simulink model "model_linear_observador"  (R2022a)
settings: Solver=VariableStepAuto  StartTime=0  StopTime=100  RelTol=1e-3
values from neighbouring files (symbols this model uses):
  A = [ 0 1 0  0 ... (first row only)    [ball_and_beam_pfc.m]
  amplitude_entrada = 0.05    [ball_and_beam_pfc.m]
  B = [0 ... (first row only)    [ball_and_beam_pfc.m]
  bool_degrau = 1    [ball_and_beam_pfc.m]
  C = [0 0 1 0]    [ball_and_beam_pfc.m]
  k_seguimento = K_nulo(1:4)    [ball_and_beam_pfc.m]
  ki_seguimento = K_nulo(5)    [ball_and_beam_pfc.m]
  L = 0.425    [ball_and_beam_pfc.m]    (also in nonlinear_ball_and_beam.m)
  L_observer = inv(T)*Lchp    [ball_and_beam_pfc.m]
libraries: vrlib x3
settings Model: Creator=Notebook_Artur  LastModifiedBy=Notebook_Artur

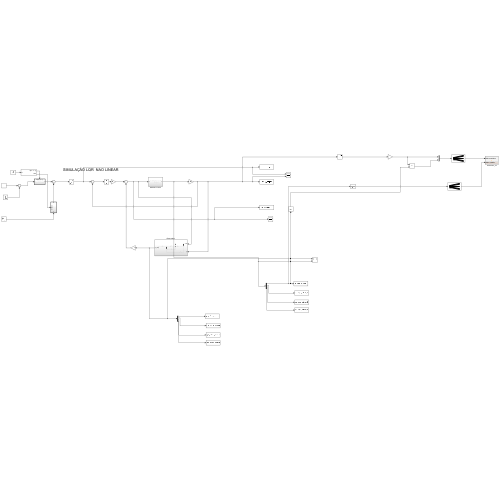
[thumbnail: Simulink's stored preview of the top-level diagram]
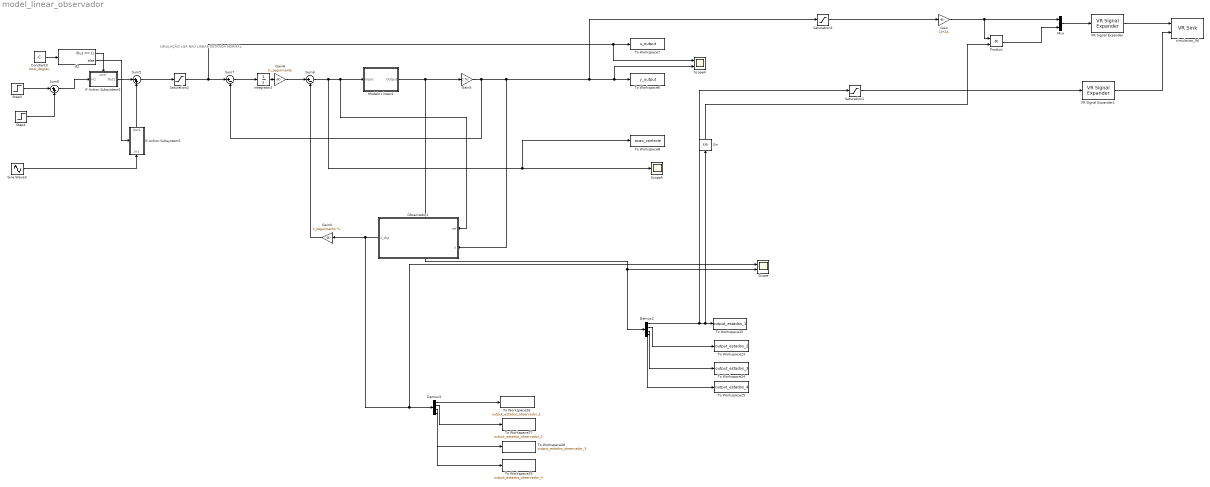
== system model_linear_observador ==
  note: SIMULAÇÃO LQR NAO LINEAR ENTRADA NORMAL
  Constant3 : Constant  Value=bool_degrau
  Demux2 : Demux
  Demux3 : Demux
  Gain : Gain  Gain=13*2/L
  Gain4 : Gain  Gain=k_seguimento  Multiplication=Matrix(K*u)
  Gain5 : Gain  Gain=C  Multiplication=Matrix(K*u)
  Gain6 : Gain  Gain=ki_seguimento
  If Action Subsystem5 : Subsystem  TreatAsAtomicUnit=on
  If Action Subsystem6 : Subsystem  TreatAsAtomicUnit=on
  If2 : If  IfExpression=u1 == 1
  Integrator2 : Integrator
  Modelo Linear2 : Subsystem
  Mux : Mux  Inputs=2
  Observador1 : Subsystem
  Product : Product
  Saturation1 : Saturate  UpperLimit=0.8  LowerLimit=-0.8
  Saturation2 : Saturate  UpperLimit=L/2  LowerLimit=-L/2
  Saturation3 : Saturate  UpperLimit=L/2  LowerLimit=0
  Scope : Scope  NumInputPorts=2
  Scope4 : Scope  NumInputPorts=2
  Scope5 : Scope
  Sin : Trigonometry
  Sine Wave3 : Sin  Amplitude=amplitude_entrada  Frequency=0.1  SampleTime=0
  Step3 : Step  After=amplitude_entrada  SampleTime=0
  Step4 : Step  Time=100  After=-2*amplitude_entrada  SampleTime=0
  Sum5 : Sum  Inputs=|++
  Sum6 : Sum  Inputs=|+-
  Sum7 : Sum  Inputs=|+-
  Sum8 : Sum  Inputs=|++
  To Workspace15 : ToWorkspace  VariableName=output_estados_1  SaveFormat=Timeseries  SampleTime=-1
  To Workspace23 : ToWorkspace  VariableName=output_estados_2  SaveFormat=Timeseries  SampleTime=-1
  To Workspace24 : ToWorkspace  VariableName=output_estados_3  SaveFormat=Timeseries  SampleTime=-1
  To Workspace25 : ToWorkspace  VariableName=output_estados_4  SaveFormat=Timeseries  SampleTime=-1
  To Workspace26 : ToWorkspace  VariableName=output_estados_observador_1  SaveFormat=Timeseries  SampleTime=-1
  To Workspace27 : ToWorkspace  VariableName=output_estados_observador_2  SaveFormat=Timeseries  SampleTime=-1
  To Workspace28 : ToWorkspace  VariableName=output_estados_observador_3  SaveFormat=Timeseries  SampleTime=-1
  To Workspace29 : ToWorkspace  VariableName=output_estados_observador_4  SaveFormat=Timeseries  SampleTime=-1
  To Workspace6 : ToWorkspace  VariableName=y_output  SaveFormat=Timeseries  SampleTime=-1
  To Workspace7 : ToWorkspace  VariableName=u_output  SaveFormat=Timeseries  SampleTime=-1
  To Workspace8 : ToWorkspace  VariableName=acao_controle  SaveFormat=Timeseries  SampleTime=-1
  VR Signal Expander : vrlib/VR Signal Expander  outwidth=3  outidx=[1 3]
  VR Signal Expander1 : vrlib/VR Signal Expander  outwidth=4  outidx=[4]
  simulacao_3d : vrlib/VR Sink  InstantiateOnLoad=on  SampleTime=0.1  ViewEnable=on  RemoteChange=off  RemoteView=off  FieldsWritten=Ball.translation.3.1.1.double#beam.rotation.4.1.1.double  WorldFileName=3d_ball_and_beam4.x3d  AutoView=on  VideoDimensions=[]  AllowVariableSize=off
  wires:
  If Action Subsystem6/1(Out1) -> Sum5/1
  Demux2/2 -> To Workspace23/1
  Demux3/2 -> To Workspace27/1
  Integrator2/1 -> Gain6/1
  If2/2 -> If Action Subsystem5/Action
  Demux2/3 -> To Workspace24/1
  Demux3/4 -> To Workspace29/1
  Demux3/3 -> To Workspace28/1
  If2/1 -> If Action Subsystem6/Action
  Modelo Linear2/1(Output) -> Gain5/1, Demux2/1, Scope/2
  Gain6/1 -> Sum6/1
  If Action Subsystem5/1(Out1) -> Sum5/2
  Demux2/4 -> To Workspace25/1
  Sum5/1 -> Saturation2/1
  Observador1/1(x_chp) -> Scope/1, Demux3/1, Gain4/1
  Sine Wave3/1 -> If Action Subsystem5/1(In1)
  Sum8/1 -> If Action Subsystem6/1(In1)
  Saturation2/1 -> To Workspace7/1, Scope4/1, Sum7/1
  Sum6/1 -> To Workspace8/1, Scope5/1, Observador1/1(ref), Modelo Linear2/1(Input)
  Constant3/1 -> If2/1
  Gain4/1 -> Sum6/2
  Step4/1 -> Sum8/2
  Sum7/1 -> Integrator2/1
  Step3/1 -> Sum8/1
  Demux3/1 -> To Workspace26/1
  Demux2/1 -> Sin/1, To Workspace15/1, Saturation1/1
  VR Signal Expander/1 -> simulacao_3d/1
  VR Signal Expander1/1 -> simulacao_3d/2
  Product/1 -> Mux/2
  Gain/1 -> Product/1, Mux/1
  Mux/1 -> VR Signal Expander/1
  Sin/1 -> Product/2
  Gain5/1 -> Saturation3/1, Scope4/2, To Workspace6/1, Observador1/2(y), Sum7/2
  Saturation1/1 -> VR Signal Expander1/1
  Saturation3/1 -> Gain/1

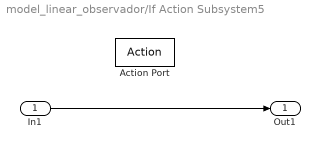
== system model_linear_observador/If Action Subsystem5 ==
  In1 : Inport
  Action Port : ActionPort  ActionPortLabel=else
  Out1 : Outport
  wires:
  In1/1 -> Out1/1

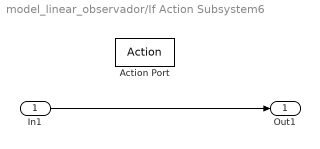
== system model_linear_observador/If Action Subsystem6 ==
  In1 : Inport
  Action Port : ActionPort  ActionPortLabel=if(u1 == 1)
  Out1 : Outport
  wires:
  In1/1 -> Out1/1

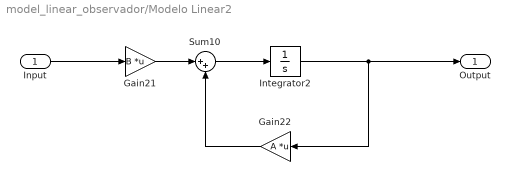
== system model_linear_observador/Modelo Linear2 ==
  Input : Inport
  Gain21 : Gain  Gain=B  Multiplication=Matrix(K*u)
  Gain22 : Gain  Gain=A  Multiplication=Matrix(K*u)
  Integrator2 : Integrator
  Sum10 : Sum  Inputs=|++
  Output : Outport
  wires:
  Input/1 -> Gain21/1
  Gain22/1 -> Sum10/2
  Integrator2/1 -> Output/1, Gain22/1
  Gain21/1 -> Sum10/1
  Sum10/1 -> Integrator2/1

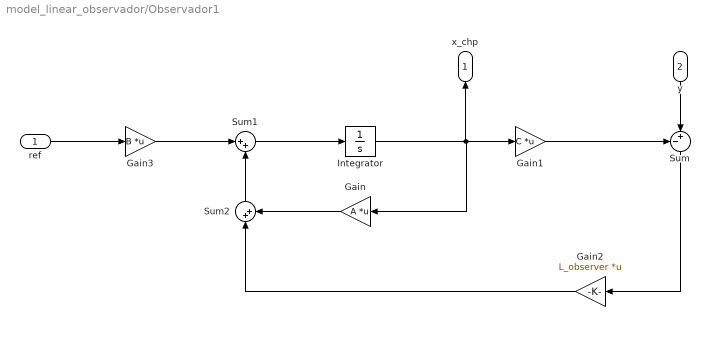
== system model_linear_observador/Observador1 ==
  ref : Inport
  y : Inport  Port=2
  Gain : Gain  Gain=A  Multiplication=Matrix(K*u)
  Gain1 : Gain  Gain=C  Multiplication=Matrix(K*u)
  Gain2 : Gain  Gain=L_observer  Multiplication=Matrix(K*u)
  Gain3 : Gain  Gain=B  Multiplication=Matrix(K*u)
  Integrator : Integrator
  Sum : Sum  Inputs=-+|
  Sum1 : Sum  Inputs=|++
  Sum2 : Sum  Inputs=|++
  x_chp : Outport
  wires:
  Integrator/1 -> x_chp/1, Gain1/1, Gain/1
  Sum/1 -> Gain2/1
  Gain1/1 -> Sum/1
  Gain/1 -> Sum2/2
  y/1 -> Sum/2
  Sum2/1 -> Sum1/2
  Gain2/1 -> Sum2/1
  Sum1/1 -> Integrator/1
  ref/1 -> Gain3/1
  Gain3/1 -> Sum1/1
